simulink model "Dummy_Subsystem"  (R2025b)
settings: Solver=VariableStepAuto  StartTime=0.0  StopTime=10.0  RelTol=1e-3
settings Model: Creator=georg  LastModifiedBy=georg

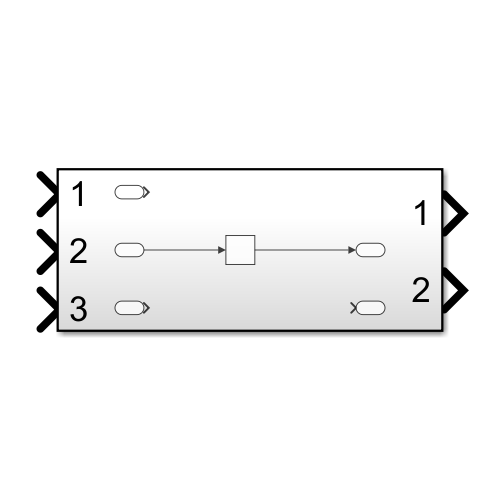
[thumbnail: Simulink's stored preview of the top-level diagram]
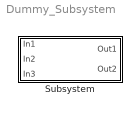
== system Dummy_Subsystem ==
  Subsystem : Subsystem

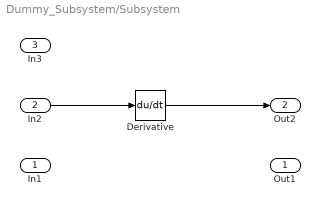
== system Dummy_Subsystem/Subsystem ==
  In1 : Inport
  In2 : Inport  Port=2
  In3 : Inport  Port=3
  Derivative : Derivative
  Out1 : Outport
  Out2 : Outport  Port=2
  wires:
  In2/1 -> Derivative/1
  Derivative/1 -> Out2/1
